simulink model "lab2s"  (R2020b)
settings: Solver=VariableStepAuto  StartTime=0.0  StopTime=10.0  RelTol=1e-3
values from neighbouring files (symbols this model uses):
  H2 = 17    [lab2.m]
  q10 = 4.12311    [lab2.m]
undefined symbols (not defined in the file or in its folder): A1, A2, C1, C2, dq1, h10, h20, x, y
settings Model: Creator=superstudent  LastModifiedBy=Marek
settings DataIOCC: ReturnWorkspaceOutputs=off
settings DebuggingCC: ArithmeticOperatorsInVariantConditions=warning
settings SFSimCC: SimUseLocalCustomCode=off  CustomCodeUndefinedFunction=UseInterfaceOnly
settings RTWCC: RTWUseLocalCustomCode=off
settings CodeAppCC: StateflowObjectComments=on

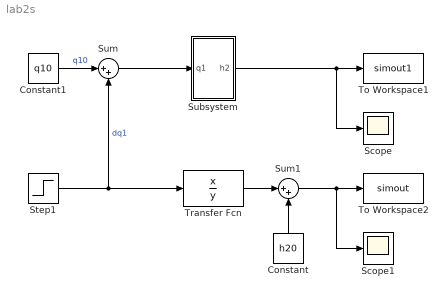
== system lab2s ==
  Constant : Constant  Value=h20
  Constant1 : Constant  Value=q10
  Scope : Scope
  Scope1 : Scope
  Step1 : Step  Time=0  After=dq1  SampleTime=0
  Subsystem : Subsystem
  Sum : Sum  Inputs=|++
  Sum1 : Sum  Inputs=|++
  To Workspace1 : ToWorkspace  VariableName=simout1  SampleTime=-1
  To Workspace2 : ToWorkspace  VariableName=simout  SampleTime=-1
  Transfer Fcn : TransferFcn  Numerator=x  Denominator=y
  wires:
  Subsystem/1(h2) -> Scope/1, To Workspace1/1
  Constant1/1 -> Sum/1  "q10"
  Sum/1 -> Subsystem/1(q1)
  Step1/1 -> Transfer Fcn/1, Sum/2  "dq1"
  Transfer Fcn/1 -> Sum1/1
  Constant/1 -> Sum1/2
  Sum1/1 -> Scope1/1, To Workspace2/1

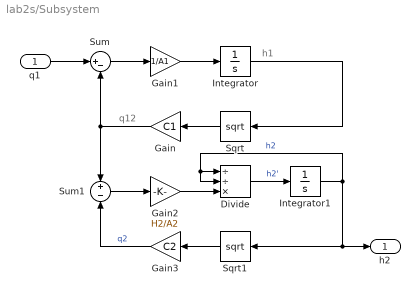
== system lab2s/Subsystem ==
  note: h1
  note: q12
  q1 : Inport
  Divide : Product  Inputs=//*
  Gain : Gain  Gain=C1
  Gain1 : Gain  Gain=1/A1
  Gain2 : Gain  Gain=H2/A2
  Gain3 : Gain  Gain=C2
  Integrator : Integrator  InitialCondition=h10
  Integrator1 : Integrator  InitialCondition=h20
  Sqrt : Sqrt  SaturateOnIntegerOverflow=on
  Sqrt1 : Sqrt  SaturateOnIntegerOverflow=on
  Sum : Sum  Inputs=|+-
  Sum1 : Sum  Inputs=+|-
  h2 : Outport
  wires:
  Gain/1 -> Sum1/1, Sum/2
  Sum/1 -> Gain1/1
  Sqrt1/1 -> Gain3/1
  Integrator1/1 -> h2/1, Sqrt1/1, Divide/1, Divide/2  "h2"
  Gain3/1 -> Sum1/2  "q2"
  Divide/1 -> Integrator1/1  "h2'"
  Integrator/1 -> Sqrt/1
  Sum1/1 -> Gain2/1
  Gain1/1 -> Integrator/1
  Sqrt/1 -> Gain/1
  Gain2/1 -> Divide/3
  q1/1 -> Sum/1
